simulink model "active_filter_spatial"  (R2015a)
settings: Solver=ode23t  StartTime=0.0  StopTime=1.5  FixedStep=Ts/50  MaxStep=Ts/50  RelTol=1e-3
values from neighbouring files (symbols this model uses):
  F1 = (1/N)*(1-z^-N)/(1-z^-1)    [angular_space_repetitive_control_design.m]
  Gcuz = c2d(ki/s+kp,Ts,'tustin')    [angular_space_repetitive_control_design.m]
  Gcz = -tf([7.976 6.657],[1 0.9511],pi/100)    [angular_space_repetitive_control_design.m]
  Gx = (1/(Goz))*tf([1],[1,zeros(1,rd)],pi/100)    [angular_space_repetitive_control_design.m]
  Kr = 0.3    [angular_space_repetitive_control_design.m]
  L = 1.2e-3    (= 0.0012)    [angular_space_repetitive_control_design.m]
  repe = feedback(Retz*H,Retz2,1)    [angular_space_repetitive_control_design.m]
  Rl = 1.4    [angular_space_repetitive_control_design.m]
  Ts = 1/12000    (= 8.33333333333e-05)    [angular_space_repetitive_control_design.m]
libraries: powerlib x24, powerlib_extras x5, powerlib_meascontrol x4, simulink x1
settings Model: CovModelRefEnable=off  CovSFcnEnable=off  Creator=asus  LastModifiedBy=sergi
settings SolverCC: ZeroCrossControl=EnableAll  ZeroCrossAlgorithm=Adaptive
settings DataIOCC: LimitDataPoints=off  SaveFormat=StructureWithTime
settings DebuggingCC: FcnCallInpInsideContextMsg=EnableAllAsWarning
settings HardwareCC: ProdBitPerPointer=64  ProdLargestAtomicFloat=Float  ProdIntDivRoundTo=Zero  ProdEndianess=LittleEndian  ProdHWDeviceType=Specified
settings GRTTargetCC: CombineOutputUpdateFcns=off  GRTInterface=on

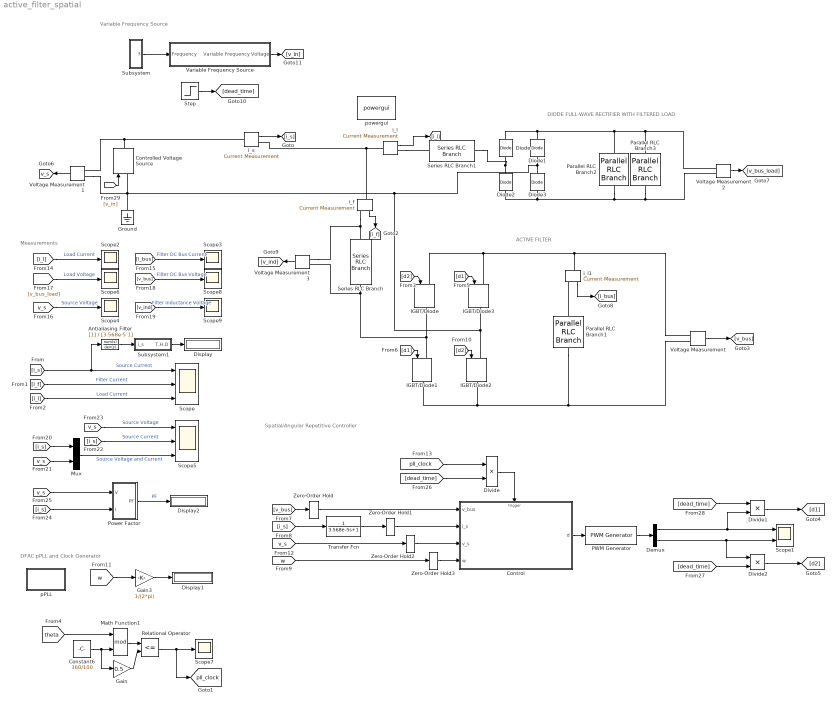
== system active_filter_spatial ==
  note: Variable Frequency Source
  note: Measurements
  note: Spatial/Angular Repetitive Controller
  note: DFAC pPLL and Clock Generator
  note: ACTIVE FILTER
  note: DIODE FULL-WAVE RECTIFIER WITH FILTERED LOAD
  Antialiasing Filter : TransferFcn  Denominator=[3.568e-5 1]
  Constant6 : Constant  Value=360/100  SampleTime=-1
  Control : Subsystem
  Controlled Voltage Source : powerlib/Electrical Sources/Controlled Voltage Source  Initialize=off  Source_Type=AC  Amplitude=0  Phase=0  Frequency=0  Measurements=None
  Demux : Demux  Outputs=2
  Diode{,1..3} (4 alike) : powerlib/Power Electronics/Diode  Ron=0.001  Lon=0  Vf=1.1  IC=0  UseSnubber=off  Rs=500  Cs=250e-9  Measurements=off
  Display : Display
  Display1 : Display
  Display2 : Display
  Divide : Product  Inputs=**
  Divide1 : Product  Inputs=**
  Divide2 : Product  Inputs=**
  Gain : Gain  Gain=0.5
  Gain3 : Gain  Gain=1/(2*pi)
  Ground : powerlib/Elements/Ground  LConnTagsString=a
  IGBT/Diode{,1..3} (4 alike) : powerlib/Power Electronics/IGBT//Diode  Ron=1e-3  Rs=1e5  Cs=inf  Measurements=off
  Math Function1 : Math  Operator=mod  SaturateOnIntegerOverflow=on
  Mux : Mux  Inputs=2
  PWM Generator : powerlib_extras/Control  Blocks/PWM Generator  GeneratorMode="1-arm  bridge (2 pulses)"  Fc=20000  Internal=off  mIndex=0.4  Freq=60  Phase=0
  Parallel RLC Branch1 : powerlib/Elements/Parallel RLC Branch  LConnTagsString=a  RConnTagsString=__new0  BranchType=RC  Resistance=8200  Inductance=1e-3  SetiL0=off  InitialCurrent=0  Capacitance=1000e-6  Setx0=on  InitialVoltage=0  Measurements=None
  Parallel RLC Branch2 : powerlib/Elements/Parallel RLC Branch  LConnTagsString=a  RConnTagsString=__new0  BranchType=RC  Resistance=1.2e3  Inductance=1e-3  SetiL0=off  InitialCurrent=0  Capacitance=470e-6  Setx0=off  InitialVoltage=30  Measurements=None
  Parallel RLC Branch3 : powerlib/Elements/Parallel RLC Branch  LConnTagsString=a  RConnTagsString=__new0  BranchType=R  Resistance=80/5  Inductance=1e-3  SetiL0=off  InitialCurrent=0  Capacitance=470e-6  Setx0=on  InitialVoltage=0  Measurements=None
  Power Factor : Subsystem
  Relational Operator : RelationalOperator  Operator=<=  OutDataTypeStr=boolean
  Scope : Scope  NumInputPorts=3
      settings: YMin=-50~-40~-7  YMax=40~35~7  SaveName=SimCurrents  DataFormat=Structure  ScrollMode=on
  Scope1 : Scope  NumInputPorts=2
      settings: YMin=-0.125~-0.125  YMax=1.125~1.125
  Scope{2..4,6..9} (7 alike) : Scope
      Scope2 settings: YMin=-10  YMax=10
      Scope3 settings: YMin=-10  YMax=10  SaveName=ScopeData2
      Scope4 settings: YMin=-10  YMax=10  SaveName=ScopeData3
      Scope6 settings: YMin=-10  YMax=10  SaveName=ScopeData4
      Scope7 settings: YMin=-0.225  YMax=2.025
      Scope8 settings: YMin=56.75  YMax=60.75  SaveName=ScopeData5
      Scope9 settings: YMin=-10  YMax=10  SaveName=ScopeData6
  Scope5 : Scope  NumInputPorts=3
      settings: YMin=-35~-27.5~-35  YMax=5~-2.5~5  SaveName=ScopeData7
  Series RLC Branch : powerlib/Elements/Series RLC Branch  LConnTagsString=__new0  RConnTagsString=__new0  BranchType=RL  Resistance=1.4  Inductance=1.2e-3  SetiL0=off  InitialCurrent=0  Capacitance=1e-6  Setx0=off  InitialVoltage=0  Measurements=None
  Series RLC Branch1 : powerlib/Elements/Series RLC Branch  LConnTagsString=__new0  RConnTagsString=__new0  BranchType=RL  Resistance=1.4  Inductance=1.2e-3  SetiL0=off  InitialCurrent=0  Capacitance=1e-6  Setx0=off  InitialVoltage=0  Measurements=None
  Step : Step  Time=0.15
  Subsystem : Subsystem
  Subsystem1 : Subsystem
  Transfer Fcn : TransferFcn  Denominator=[3.568e-5 1]
  Variable Frequency Source : Subsystem
  Voltage Measurement{,1..3} (4 alike) : powerlib/Measurements/Voltage Measurement  PhasorSimulation=off  OutputType=Complex  PSBequivalent=0
  Zero-Order Hold{,1..3} (4 alike) : ZeroOrderHold  SampleTime=Ts
  i_f : powerlib/Measurements/Current Measurement  PhasorSimulation=off  OutputType=Complex  PSBequivalent=0
  i_l : powerlib/Measurements/Current Measurement  PhasorSimulation=off  OutputType=Complex  PSBequivalent=0
  i_l1 : powerlib/Measurements/Current Measurement  PhasorSimulation=off  OutputType=Complex  PSBequivalent=0
  i_s : powerlib/Measurements/Current Measurement  PhasorSimulation=off  OutputType=Complex  PSBequivalent=0
  pPLL : Subsystem  SystemSampleTime=100e-6
  powergui : powerlib/powergui  Priority=1  SimulationMode=Continuous  SolverType=Tustin  SampleTime=Ts  frequency=60  SPID=off  DisableSnubberDevices=off  DisableRonSwitches=off  DisableVfSwitches=off  SwTol=0  DisplayEquations=off  Interpol=off  methode=off  Ts=10  FunctionMessages=off  echomessages=off  HookPort=off  EnableUseOfTLC=off  x0status=blocks  frequencyindice=0  Pbase=100e6  ErrMax=1e-4  Iterations=50  UnitsV=kV  UnitsW=MW  buscounter=0  RestoreLinks=warning  ResistiveCurrentMeasurement=off  Frange=[0:2:500]  Ylog=off  Xlog=on  ShowGrid=off  save=off  variable=ZData  structure=0  ZoomFFT=off  StartTime=0.0  cycles=1  DisplayStyle=1  fundamental=60  FreqAxis=off  MaxFrequency=1000  frequencyindicesteady=1  RmsSteady=1  display=off
  tag scope: pll_clock=global, v_s=global
  wires:
  i_s/1 -> [i_s]
  i_f/1 -> [i_f]
  [i_s] -> Antialiasing Filter/1, Scope/1  "Source Current"
  [i_f] -> Scope/2  "Filter Current"
  [i_l] -> Scope/3  "Load Current"
  Voltage Measurement/1 -> [v_bus]
  [v_bus] -> Zero-Order Hold/1
  Voltage Measurement1/1 -> [v_s]
  Voltage Measurement3/1 -> [v_ind]
  i_l1/1 -> [i_bus]
  i_l/1 -> [i_l]
  [d2] -> IGBT/Diode2/1
  [d1] -> IGBT/Diode3/1
  [w] -> Gain3/1
  [v_s] -> Zero-Order Hold2/1
  Zero-Order Hold/1 -> Control/1(v_bus)
  Zero-Order Hold1/1 -> Control/2(i_s)
  Zero-Order Hold2/1 -> Control/3(v_s)
  [theta] -> Math Function1/1
  Constant6/1 -> Gain/1, Math Function1/2
  Math Function1/1 -> Relational Operator/1
  Relational Operator/1 -> [pll_clock], Scope7/1
  Gain/1 -> Relational Operator/2
  PWM Generator/1 -> Demux/1
  Control/1(d) -> PWM Generator/1
  Demux/2 -> Scope1/2, Divide2/1
  Demux/1 -> Scope1/1, Divide1/2
  Subsystem1/1(T.H.D) -> Display/1
  Divide/1 -> Control/Trigger
  [dead_time] -> Divide/2
  [dead_time] -> Divide1/1
  Divide1/1 -> [d1]
  [dead_time] -> Divide2/2
  Divide2/1 -> [d2]
  [w] -> Zero-Order Hold3/1
  Zero-Order Hold3/1 -> Control/4(w)
  [pll_clock] -> Divide/1
  [d1] -> IGBT/Diode1/1
  [d2] -> IGBT/Diode/1
  [i_s] -> Transfer Fcn/1
  Transfer Fcn/1 -> Zero-Order Hold1/1
  Antialiasing Filter/1 -> Subsystem1/1(i_s)
  Gain3/1 -> Display1/1
  Voltage Measurement2/1 -> [v_bus_load]
  [i_l] -> Scope2/1  "Load Current"
  [i_bus] -> Scope3/1  "Filter DC Bus Current"
  [v_s] -> Scope4/1  "Source Voltage"
  [v_bus_load] -> Scope6/1  "Load Voltage"
  [v_bus] -> Scope8/1  "Filter DC Bus Voltage"
  [v_ind] -> Scope9/1  "Filter Inductance Voltage"
  Mux/1 -> Scope5/3  "Source Voltage and Current"
  [i_s] -> Mux/1
  [v_s] -> Mux/2
  [i_s] -> Scope5/2  "Source Current"
  [v_s] -> Scope5/1  "Source Voltage"
  [v_s] -> Power Factor/1(V)
  [i_s] -> Power Factor/2(I)
  Power Factor/1(PF) -> Display2/1  "PF"
  Step/1 -> [dead_time]
  Variable Frequency Source/1(Variable Frequency Voltage) -> [v_in]
  [v_in] -> Controlled Voltage Source/1
  Subsystem/1(f) -> Variable Frequency Source/1(Frequency)
  connections:
  Diode/RConn1 -- Parallel RLC Branch3/LConn1 -- Voltage Measurement2/LConn1 -- Parallel RLC Branch2/LConn1 -- Diode1/RConn1
  i_f/RConn1 -- Voltage Measurement3/LConn1 -- Series RLC Branch/LConn1
  i_l1/LConn1 -- IGBT/Diode3/LConn1 -- IGBT/Diode/LConn1 -- Voltage Measurement/LConn1
  Voltage Measurement/LConn2 -- IGBT/Diode1/RConn1 -- IGBT/Diode2/RConn1 -- Parallel RLC Branch1/RConn1
  Series RLC Branch/RConn1 -- Voltage Measurement3/LConn2 -- IGBT/Diode1/LConn1 -- IGBT/Diode/RConn1
  i_l/LConn1 -- i_f/LConn1 -- i_s/RConn1
  i_s/LConn1 -- Voltage Measurement1/LConn1 -- Controlled Voltage Source/RConn1
  Diode2/RConn1 -- Series RLC Branch1/LConn1 -- Diode/LConn1
  Diode3/LConn1 -- Parallel RLC Branch3/RConn1 -- Voltage Measurement2/LConn2 -- Parallel RLC Branch2/RConn1 -- Diode2/LConn1
  IGBT/Diode2/LConn1 -- IGBT/Diode3/RConn1 -- Controlled Voltage Source/LConn1 -- Ground/LConn1 -- Voltage Measurement1/LConn2 -- Diode1/LConn1 -- Diode3/RConn1
  Parallel RLC Branch1/LConn1 -- i_l1/RConn1
  i_l/RConn1 -- Series RLC Branch1/RConn1

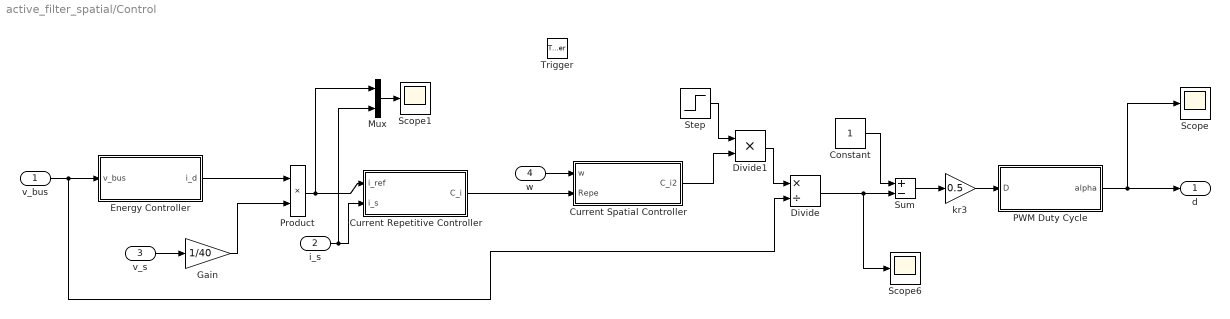
== system active_filter_spatial/Control ==
  v_bus : Inport
  i_s : Inport  Port=2
  v_s : Inport  Port=3
  w : Inport  Port=4
  Trigger : TriggerPort  TriggerType=either  PortDimensions=1
  Constant : Constant
  Current Repetitive Controller : Subsystem  SystemSampleTime=1/12000
  Current Spatial Controller : Subsystem
  Divide : Product  Inputs=*/
  Divide1 : Product  Inputs=**
  Energy Controller : Subsystem  SystemSampleTime=1/12000
  Gain : Gain  Gain=1/40
  Mux : Mux  Inputs=2
  PWM Duty Cycle : Subsystem  SystemSampleTime=1/12000
  Product : Product
  Scope : Scope
      settings: YMin=-0.84934  YMax=0.73316
  Scope1 : Scope
      settings: YMin=4.80661  YMax=19.08277  SaveName=ScopeData7
  Scope6 : Scope
      settings: YMin=4.80661  YMax=19.08277  SaveName=ScopeData6
  Step : Step  Time=0.15
  Sum : Sum  Inputs=+-
  kr3 : Gain  Gain=0.5
  d : Outport
  wires:
  Current Repetitive Controller/1(C_i) -> Current Spatial Controller/2(Repe)
  Product/1 -> Mux/1, Current Repetitive Controller/1(i_ref)
  v_bus/1 -> Divide/2, Energy Controller/1(v_bus)
  i_s/1 -> Mux/2, Current Repetitive Controller/2(i_s)
  v_s/1 -> Gain/1
  Gain/1 -> Product/2
  Constant/1 -> Sum/1
  Sum/1 -> kr3/1
  Divide/1 -> Scope6/1, Sum/2
  Energy Controller/1(i_d) -> Product/1
  Mux/1 -> Scope1/1
  kr3/1 -> PWM Duty Cycle/1(D)
  PWM Duty Cycle/1(alpha) -> d/1, Scope/1
  w/1 -> Current Spatial Controller/1(w)
  Step/1 -> Divide1/1
  Current Spatial Controller/1(C_i2) -> Divide1/2
  Divide1/1 -> Divide/1

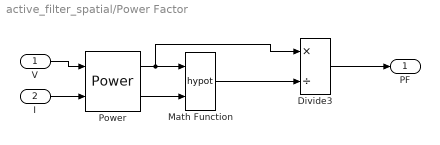
== system active_filter_spatial/Power Factor ==
  V : Inport
  I : Inport  Port=2
  Divide3 : Product  Inputs=*/
  Math Function : Math  Operator=hypot  SaturateOnIntegerOverflow=on
  Power : powerlib_meascontrol/Measurements/Power  Freq=60  Vinit=[1, 0]  Iinit=[1, 0]  Ts=0
  PF : Outport
  wires:
  Power/1 -> Divide3/1, Math Function/1
  I/1 -> Power/2
  Math Function/1 -> Divide3/2
  Divide3/1 -> PF/1
  V/1 -> Power/1
  Power/2 -> Math Function/2

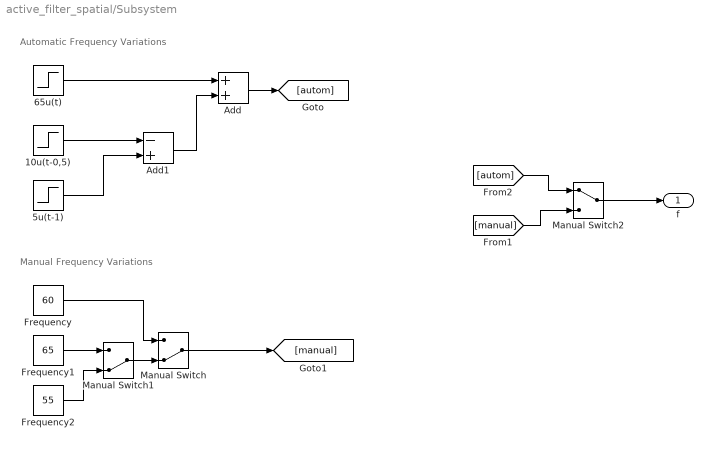
== system active_filter_spatial/Subsystem ==
  note: Manual Frequency Variations
  note: Automatic Frequency Variations
  10u(t-0,5) : Step  Time=0.5  After=10  SampleTime=0
  5u(t-1) : Step  After=5  SampleTime=0
  65u(t) : Step  Time=0  After=65  SampleTime=0
  Add : Sum
  Add1 : Sum  Inputs=-+
  Frequency : Constant  Value=60
  Frequency1 : Constant  Value=65
  Frequency2 : Constant  Value=55
  Manual Switch : ManualSwitch  CurrentSetting=0
  Manual Switch1 : ManualSwitch  CurrentSetting=0
  Manual Switch2 : ManualSwitch
  f : Outport
  wires:
  65u(t)/1 -> Add/1
  10u(t-0,5)/1 -> Add1/1
  5u(t-1)/1 -> Add1/2
  Add1/1 -> Add/2
  Manual Switch/1 -> [manual]
  Manual Switch1/1 -> Manual Switch/2
  Frequency/1 -> Manual Switch/1
  Frequency1/1 -> Manual Switch1/1
  Frequency2/1 -> Manual Switch1/2
  Add/1 -> [autom]
  [autom] -> Manual Switch2/1
  [manual] -> Manual Switch2/2
  Manual Switch2/1 -> f/1

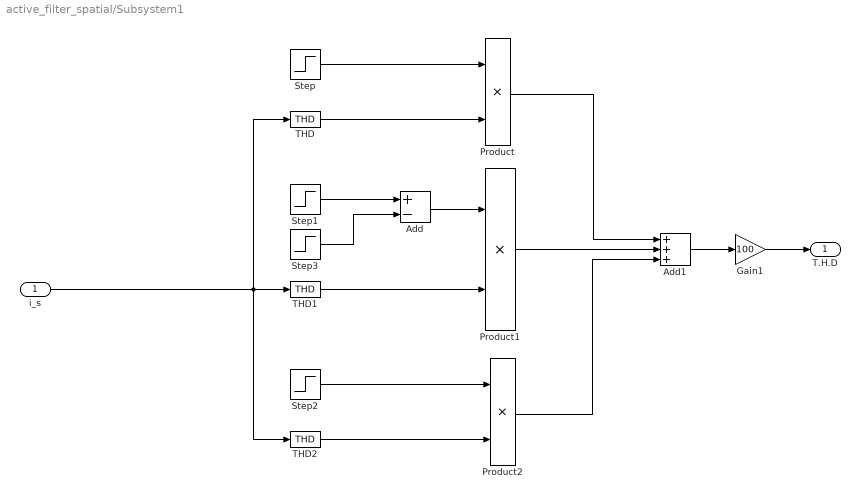
== system active_filter_spatial/Subsystem1 ==
  i_s : Inport
  Add : Sum  Inputs=+-
  Add1 : Sum  Inputs=+++
  Gain1 : Gain  Gain=100
  Product : Product
  Product1 : Product
  Product2 : Product
  Step : Step  Time=0.5  Before=1  After=0  SampleTime=0
  Step1 : Step  Time=0.5  SampleTime=0
  Step2 : Step  SampleTime=0
  Step3 : Step  SampleTime=0
  THD : powerlib_meascontrol/Measurements/THD  Freq=65  Ts=0
  THD1 : powerlib_meascontrol/Measurements/THD  Freq=55  Ts=0
  THD2 : powerlib_meascontrol/Measurements/THD  Freq=60  Ts=0
  T.H.D : Outport
  wires:
  Step/1 -> Product/1
  THD/1 -> Product/2
  THD1/1 -> Product1/2
  Step2/1 -> Product2/1
  Step1/1 -> Add/1
  Step3/1 -> Add/2
  Add/1 -> Product1/1
  i_s/1 -> THD2/1, THD/1, THD1/1
  THD2/1 -> Product2/2
  Product/1 -> Add1/1
  Product1/1 -> Add1/2
  Product2/1 -> Add1/3
  Add1/1 -> Gain1/1
  Gain1/1 -> T.H.D/1

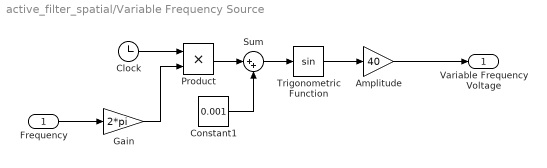
== system active_filter_spatial/Variable Frequency Source ==
  Frequency : Inport
  Amplitude : Gain  Gain=40
  Clock : Clock
  Constant1 : Constant  Value=0.001
  Gain : Gain  Gain=2*pi
  Product : Product
  Sum : Sum  Inputs=|++
  Trigonometric Function : Trigonometry
  Variable Frequency Voltage : Outport
  wires:
  Clock/1 -> Product/1
  Sum/1 -> Trigonometric Function/1
  Constant1/1 -> Sum/2
  Product/1 -> Sum/1
  Trigonometric Function/1 -> Amplitude/1
  Amplitude/1 -> Variable Frequency Voltage/1
  Frequency/1 -> Gain/1
  Gain/1 -> Product/2

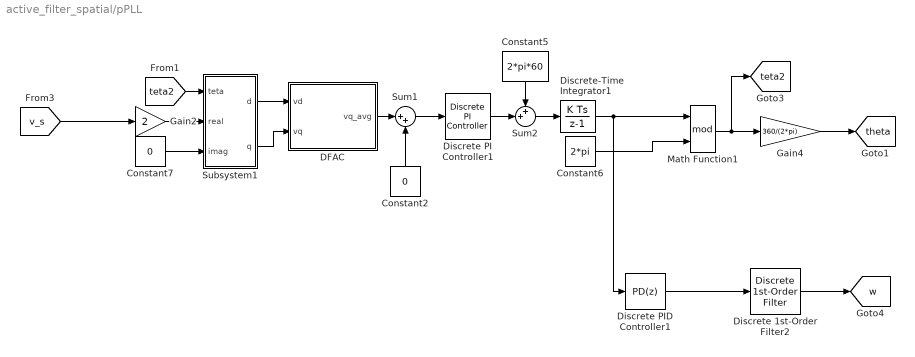
== system active_filter_spatial/pPLL ==
  Constant2 : Constant  Value=0
  Constant5 : Constant  Value=2*pi*60
  Constant6 : Constant  Value=2*pi  SampleTime=-1
  Constant7 : Constant  Value=0
  DFAC : Subsystem
  Discrete 1st-Order Filter2 : powerlib_extras/Discrete  Control Blocks/Discrete 1st-Order Filter  FilterType=Lowpass  Tc=20e-3  Ts=1/600000  Initialize=off  Vac_Init=[0.8 -25 55]  Vdc_Init=-0.4  PlotResponse=off  param1=[1 500 0.1]
  Discrete PI Controller1 : powerlib_extras/Discrete  Control Blocks/Discrete PI Controller  Kp=43.76*pi  Ki=(43.76*pi*43.76*pi)/2.4  Par_Limits=[1e6 -1e6]  Init=0  Ts=1/600000
  Discrete PID Controller1 : simulink/Continuous/PID Controller  Controller=PD  TimeDomain=Discrete-time  SampleTime=1/600000  IntegratorMethod=Forward Euler  FilterMethod=Forward Euler  Form=Parallel  UseFilter=on  ControllerParametersSource=internal  P=0  I=1  D=1  N=2500  InitialConditionSource=internal  InitialConditionForIntegrator=0  InitialConditionForFilter=0  ExternalReset=none  LimitOutput=off  UpperSaturationLimit=inf  LowerSaturationLimit=-inf  LinearizeAsGain=off  AntiWindupMode=none  Kb=1  TrackingMode=off  Kt=1  PParamMin=[]  PParamMax=[]  IParamMin=[]  IParamMax=[]  DParamMin=[]  DParamMax=[]  NParamMin=[]  NParamMax=[]  KbParamMin=[]  KbParamMax=[]  KtParamMin=[]  KtParamMax=[]  POutMin=[]  POutMax=[]  IOutMin=[]  IOutMax=[]  DOutMin=[]  DOutMax=[]  NOutMin=[]  NOutMax=[]  KbOutMin=[]  KbOutMax=[]  KtOutMin=[]  KtOutMax=[]  IntegratorOutMin=[]  IntegratorOutMax=[]  FilterOutMin=[]  FilterOutMax=[]  SumOutMin=[]  SumOutMax=[]  SumI1OutMin=[]  SumI1OutMax=[]  SumI2OutMin=[]  SumI2OutMax=[]  SumI3OutMin=[]  SumI3OutMax=[]  SumDOutMin=[]  SumDOutMax=[]  SaturationOutMin=[]  SaturationOutMax=[]  IntegratorContinuousStateAttributes=''  IntegratorStateMustResolveToSignalObject=off  IntegratorRTWStateStorageClass=Auto  FilterContinuousStateAttributes=''  FilterStateMustResolveToSignalObject=off  FilterRTWStateStorageClass=Auto  DifferentiatorICPrevScaledInput=0  DifferentiatorOutMin=[]  DifferentiatorOutMax=[]
  Discrete-Time Integrator1 : DiscreteIntegrator  SampleTime=1/600000
  Gain2 : Gain  Gain=2
  Gain4 : Gain  Gain=360/(2*pi)
  Math Function1 : Math  Operator=mod  SaturateOnIntegerOverflow=on
  Subsystem1 : Subsystem
  Sum1 : Sum  Inputs=|++
  Sum2 : Sum  Inputs=++|
  tag scope: teta2=global, theta=global, w=global
  wires:
  Constant2/1 -> Sum1/2
  Constant5/1 -> Sum2/1
  Discrete PI Controller1/1 -> Sum2/2
  Sum2/1 -> Discrete-Time Integrator1/1
  Math Function1/1 -> Gain4/1, [teta2]
  Gain2/1 -> Subsystem1/2(real)
  Constant7/1 -> Subsystem1/3(imag)
  DFAC/1(vq_avg) -> Sum1/1
  Subsystem1/1(d) -> DFAC/1(vd)
  Subsystem1/2(q) -> DFAC/2(vq)
  Sum1/1 -> Discrete PI Controller1/1
  Discrete-Time Integrator1/1 -> Math Function1/1, Discrete PID Controller1/1
  Constant6/1 -> Math Function1/2
  [teta2] -> Subsystem1/1(teta)
  Discrete 1st-Order Filter2/1 -> [w]
  [v_s] -> Gain2/1
  Gain4/1 -> [theta]
  Discrete PID Controller1/1 -> Discrete 1st-Order Filter2/1

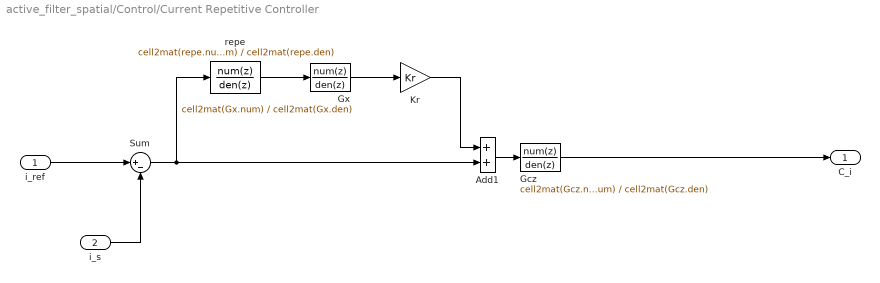
== system active_filter_spatial/Control/Current Repetitive Controller ==
  i_ref : Inport
  i_s : Inport  Port=2
  Add1 : Sum
  Gcz : DiscreteTransferFcn  Numerator=cell2mat(Gcz.num)  Denominator=cell2mat(Gcz.den)
  Gx : DiscreteTransferFcn  Numerator=cell2mat(Gx.num)  Denominator=cell2mat(Gx.den)
  Kr : Gain  Gain=Kr
  Sum : Sum  Inputs=|+-
  repe : DiscreteTransferFcn  Numerator=cell2mat(repe.num)  Denominator=cell2mat(repe.den)
  C_i : Outport
  wires:
  i_ref/1 -> Sum/1
  i_s/1 -> Sum/2
  Kr/1 -> Add1/1
  Add1/1 -> Gcz/1
  Sum/1 -> Add1/2, repe/1
  Gcz/1 -> C_i/1
  repe/1 -> Gx/1
  Gx/1 -> Kr/1

== system active_filter_spatial/Control/Current Spatial Controller ==
  w : Inport
  Repe : Inport  Port=2
  Plant Precompensation : Subsystem
  C_i2 : Outport
  wires:
  w/1 -> Plant Precompensation/2(omega)
  Plant Precompensation/1("y ") -> C_i2/1
  Repe/1 -> Plant Precompensation/1(x)

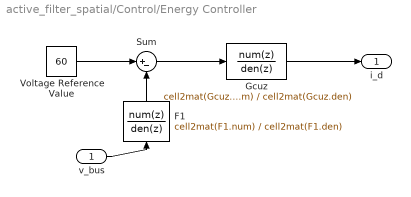
== system active_filter_spatial/Control/Energy Controller ==
  v_bus : Inport
  F1 : DiscreteTransferFcn  Numerator=cell2mat(F1.num)  Denominator=cell2mat(F1.den)
  Gcuz : DiscreteTransferFcn  Numerator=cell2mat(Gcuz.num)  Denominator=cell2mat(Gcuz.den)
  Sum : Sum  Inputs=|+-
  Voltage Reference Value : Constant  Value=60
  i_d : Outport
  wires:
  Voltage Reference Value/1 -> Sum/1
  v_bus/1 -> F1/1
  Sum/1 -> Gcuz/1
  Gcuz/1 -> i_d/1
  F1/1 -> Sum/2

== system active_filter_spatial/Control/PWM Duty Cycle ==
  D : Inport
  Fcn : Fcn  Expr=2*u-1
  Scope : Scope
      settings: YMin=-10  YMax=10  SaveName=ScopeData4
  Scope1 : Scope
      settings: YMin=-202163794169621330000000.00000  YMax=338506244278945980000000.00000  SaveName=ScopeData5
  alpha : Outport
  wires:
  Fcn/1 -> Scope1/1, alpha/1
  D/1 -> Scope/1, Fcn/1

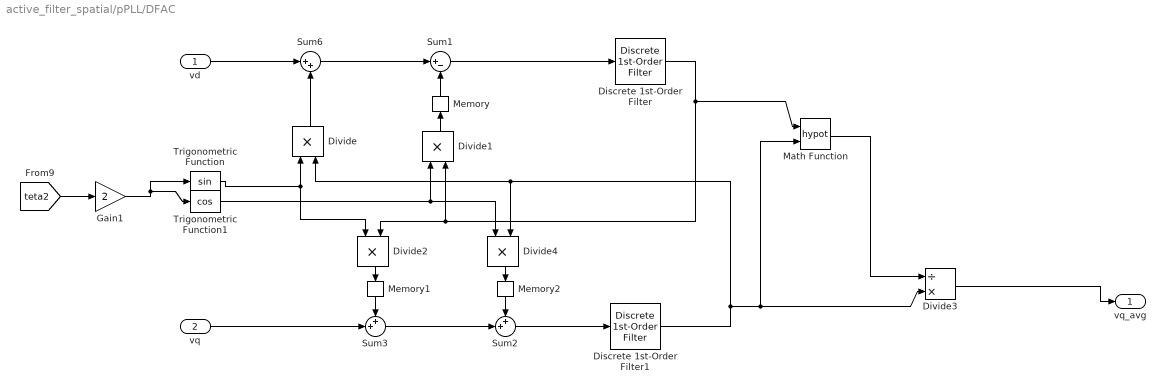
== system active_filter_spatial/pPLL/DFAC ==
  vd : Inport
  vq : Inport  Port=2
  Discrete 1st-Order Filter : powerlib_extras/Discrete  Control Blocks/Discrete 1st-Order Filter  FilterType=Lowpass  Tc=1/(105.024*pi)  Ts=1/600000  Initialize=off  Vac_Init=[0.8 -25 60]  Vdc_Init=-0.4  PlotResponse=off  param1=[1 500 0.1]
  Discrete 1st-Order Filter1 : powerlib_extras/Discrete  Control Blocks/Discrete 1st-Order Filter  FilterType=Lowpass  Tc=1/(105.024*pi)  Ts=1/600000  Initialize=off  Vac_Init=[0.8 -25 60]  Vdc_Init=-0.4  PlotResponse=off  param1=[1 500 0.1]
  Divide{,1..2,4} (4 alike) : Product  Inputs=**
  Divide3 : Product  Inputs=/*
  Gain1 : Gain  Gain=2
  Math Function : Math  Operator=hypot  SaturateOnIntegerOverflow=on
  Memory : Memory
  Memory1 : Memory
  Memory2 : Memory
  Sum1 : Sum  Inputs=|+-
  Sum2 : Sum  Inputs=++|
  Sum3 : Sum  Inputs=++|
  Sum6 : Sum  Inputs=|++
  Trigonometric Function : Trigonometry
  Trigonometric Function1 : Trigonometry  Operator=cos
  vq_avg : Outport
  wires:
  Memory2/1 -> Sum2/1
  Divide4/1 -> Memory2/1
  Memory1/1 -> Sum3/1
  Divide2/1 -> Memory1/1
  Memory/1 -> Sum1/2
  Divide3/1 -> vq_avg/1
  Math Function/1 -> Divide3/1
  Gain1/1 -> Trigonometric Function1/1, Trigonometric Function/1
  Sum2/1 -> Discrete 1st-Order Filter1/1
  Discrete 1st-Order Filter/1 -> Math Function/1, Divide1/2, Divide2/2
  Trigonometric Function1/1 -> Divide4/1, Divide1/1
  Trigonometric Function/1 -> Divide2/1, Divide/1
  [teta2] -> Gain1/1
  Sum3/1 -> Sum2/2
  vq/1 -> Sum3/2
  Sum1/1 -> Discrete 1st-Order Filter/1
  vd/1 -> Sum6/1
  Discrete 1st-Order Filter1/1 -> Divide3/2, Math Function/2, Divide4/2, Divide/2
  Divide1/1 -> Memory/1
  Sum6/1 -> Sum1/1
  Divide/1 -> Sum6/2

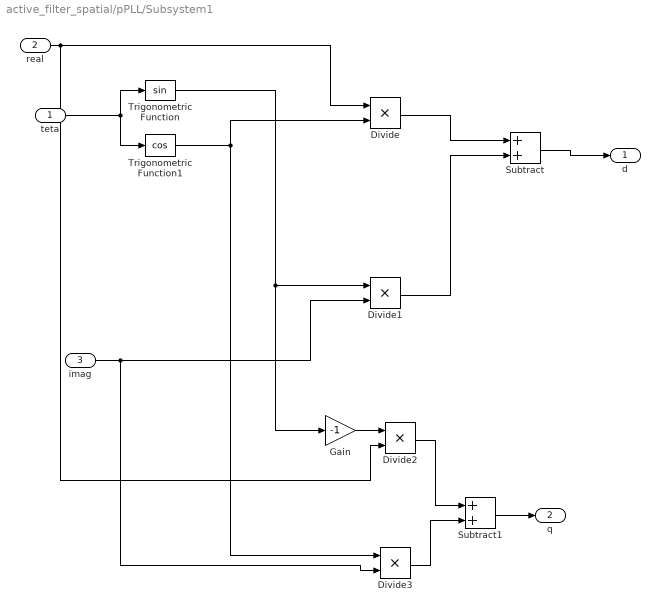
== system active_filter_spatial/pPLL/Subsystem1 ==
  teta : Inport
  real : Inport  Port=2
  imag : Inport  Port=3
  Divide{,1..3} (4 alike) : Product  Inputs=**
  Gain : Gain  Gain=-1
  Subtract : Sum
  Subtract1 : Sum
  Trigonometric Function : Trigonometry
  Trigonometric Function1 : Trigonometry  Operator=cos
  d : Outport
  q : Outport  Port=2
  wires:
  Subtract/1 -> d/1
  Subtract1/1 -> q/1
  Trigonometric Function/1 -> Divide1/1, Gain/1
  Divide3/1 -> Subtract1/2
  Divide2/1 -> Subtract1/1
  Gain/1 -> Divide2/1
  Divide1/1 -> Subtract/2
  Divide/1 -> Subtract/1
  imag/1 -> Divide3/2, Divide1/2
  Trigonometric Function1/1 -> Divide3/1, Divide/2
  real/1 -> Divide2/2, Divide/1
  teta/1 -> Trigonometric Function1/1, Trigonometric Function/1

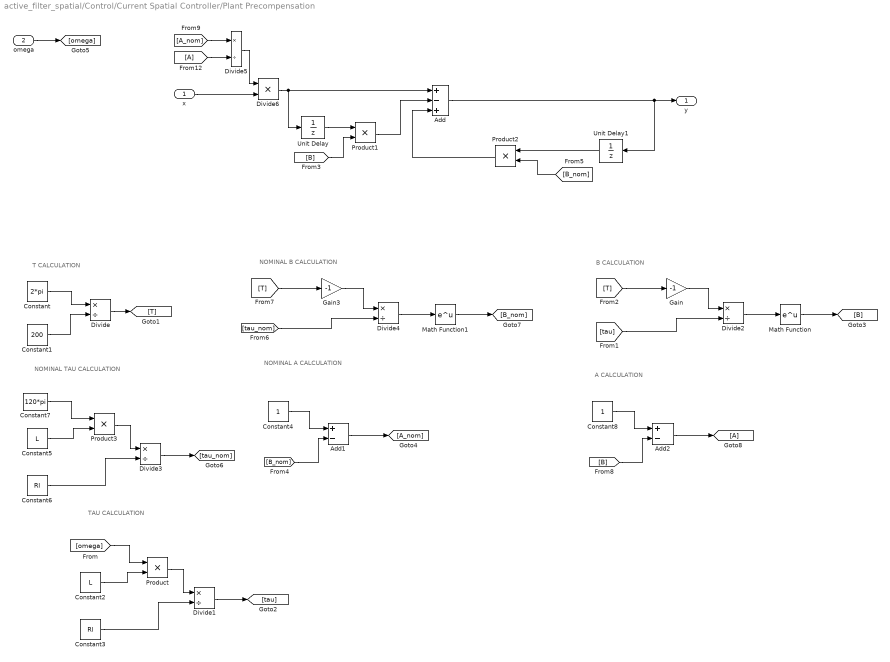
== system active_filter_spatial/Control/Current Spatial Controller/Plant Precompensation ==
  note: A CALCULATION
  note: B CALCULATION
  note: NOMINAL A CALCULATION
  note: NOMINAL B CALCULATION
  note: T CALCULATION
  note: TAU CALCULATION
  note: NOMINAL TAU CALCULATION
  x : Inport
  omega : Inport  Port=2
  Add : Sum  Inputs=+-+
  Add1 : Sum  Inputs=+-
  Add2 : Sum  Inputs=+-
  Constant : Constant  Value=2*pi
  Constant1 : Constant  Value=200
  Constant2 : Constant  Value=L
  Constant3 : Constant  Value=Rl
  Constant4 : Constant
  Constant5 : Constant  Value=L
  Constant6 : Constant  Value=Rl
  Constant7 : Constant  Value=120*pi
  Constant8 : Constant
  Divide{,1..5} (6 alike) : Product  Inputs=*/
  Divide6 : Product  Inputs=**
  Gain : Gain  Gain=-1
  Gain3 : Gain  Gain=-1
  Math Function : Math  SaturateOnIntegerOverflow=on
  Math Function1 : Math  SaturateOnIntegerOverflow=on
  Product{,1..3} (4 alike) : Product
  Unit Delay : UnitDelay  SampleTime=-1
  Unit Delay1 : UnitDelay  SampleTime=-1
  "y " : Outport
  wires:
  x/1 -> Divide6/2
  Add/1 -> Unit Delay1/1, "y "/1
  Constant/1 -> Divide/1
  Constant1/1 -> Divide/2
  Divide/1 -> [T]
  [omega] -> Product/1
  Constant2/1 -> Product/2
  Product/1 -> Divide1/1
  Constant3/1 -> Divide1/2
  Divide1/1 -> [tau]
  [T] -> Gain/1
  Gain/1 -> Divide2/1
  [tau] -> Divide2/2
  Divide2/1 -> Math Function/1
  Math Function/1 -> [B]
  Constant4/1 -> Add1/1
  [B_nom] -> Add1/2
  Add1/1 -> [A_nom]
  Unit Delay/1 -> Product1/1
  Product1/1 -> Add/2
  omega/1 -> [omega]
  Product2/1 -> Add/3
  [B_nom] -> Product2/2
  Unit Delay1/1 -> Product2/1
  Constant7/1 -> Product3/1
  Constant5/1 -> Product3/2
  Product3/1 -> Divide3/1
  Constant6/1 -> Divide3/2
  Divide3/1 -> [tau_nom]
  [T] -> Gain3/1
  Gain3/1 -> Divide4/1
  [tau_nom] -> Divide4/2
  Divide4/1 -> Math Function1/1
  Math Function1/1 -> [B_nom]
  Constant8/1 -> Add2/1
  [B] -> Add2/2
  Add2/1 -> [A]
  Divide6/1 -> Unit Delay/1, Add/1
  [B] -> Product1/2
  [A_nom] -> Divide5/1
  [A] -> Divide5/2
  Divide5/1 -> Divide6/1
